simulink model "TestIMU_Multiple"  (R2016b)
settings: Solver=VariableStepAuto  StartTime=0.0  StopTime=10.0  RelTol=1e-3
settings Model: Creator=rega0051  LastModifiedBy=katiekwiz

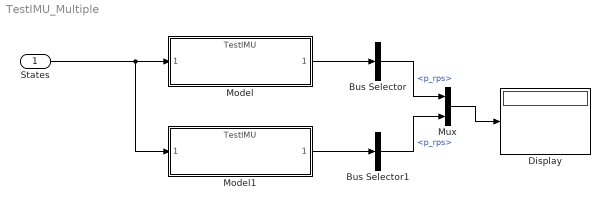
== system TestIMU_Multiple ==
  "States " : Inport  OutDataTypeStr=Bus: States
  Bus Selector : BusSelector  OutputSignals=p_rps
  Bus Selector1 : BusSelector  OutputSignals=p_rps
  Display : Display
  Model : ModelReference  ModelNameDialog=TestIMU.slx  ParameterArgumentNames=sens  ParameterArgumentValues=Param1  SimulationMode=Normal  ModelReferenceVersion=1.9
  Model1 : ModelReference  ModelNameDialog=TestIMU.slx  ParameterArgumentNames=sens  ParameterArgumentValues=Param2  SimulationMode=Normal  ModelReferenceVersion=1.9
  Mux : Mux  Inputs=2
  wires:
  "States "/1 -> Model1/1, Model/1
  Model/1 -> Bus Selector/1
  Model1/1 -> Bus Selector1/1
  Bus Selector/1 -> Mux/1  "<p_rps>"
  Bus Selector1/1 -> Mux/2  "<p_rps>"
  Mux/1 -> Display/1
